simulink model "SISO_up_plant_PI_LEAD_2019a"  (R2023b)
settings: Solver=ode4  StartTime=0.0  StopTime=sim_time  FixedStep=STEP_SIZE  RelTol=1e-3  EnableMultiTasking=on
values from neighbouring files (symbols this model uses):
  A = [0 1 0 ... (first row only)    [LuenbergerObserver.m]    (also in SISO_up_plant_init.m = 0.01)
  a2 = 110544599.2    [params_aaa_elb.mat]
  b2 = 0.0564    [params_aaa_elb.mat]
  bias = -0.02    [SISO_up_plant_init.m]
  cm2m = 0.01    [params_aaa_elb.mat]
  f2 = -880    [params_aaa_elb.mat]
  freq = 1    [SISO_up_plant_init.m]
  g = 9.816    [params_aaa_elb.mat]
  g2 = 3.66    [params_aaa_elb.mat]
  h2 = 2e-05    [params_aaa_elb.mat]
  Kc_neg = 0.114    [params_aaa_elb.mat]
  Kc_pos = 0.145    [params_aaa_elb.mat]
  Kp = 6.4782e+05    (= 647820)    [SISO_up_plant_init.m]
  Kv = 5.8    [params_aaa_elb.mat]
  m = 0.1203    [params_aaa_elb.mat]
  N = 4    [params_aaa_elb.mat]
  ref = -0.02    [SISO_up_plant_init.m]
  SatLimLower = -14000    [params_aaa_elb.mat]
  SatLimUpper = 14000    [params_aaa_elb.mat]
  yc = 0.129    [params_aaa_elb.mat]
undefined symbols (not defined in the file or in its folder): den_CD, den_CPI, num_CD, num_CPI
settings Model: SimulationMode=external  Creator=s214680  LastModifiedBy=amaln
settings SolverCC: AlgebraicLoopSolver=TrustRegion
settings HardwareCC: ProdBitPerLong=64  ProdHWDeviceType=Intel->x86-64 (Linux 64)
settings SFSimCC: CustomCodeUndefinedFunction=UseInterfaceOnly
settings RTWCC: Description=Simulink Desktop Real-Time  SystemTargetFile=sldrt.tlc  TemplateMakefile=sldrt.tmf  RTWCompilerOptimization=on
settings CodeAppCC: MaxIdLength=95
settings SimulinkDesktopRealTimeCC: TargetLibSuffix=_sldrt.a  TargetPreCompLibLocation=C:\Program Files\MATLAB\R2023b\toolbox\sldrt\lib\win64  TargetLangStandard=C89/C90 (ANSI)

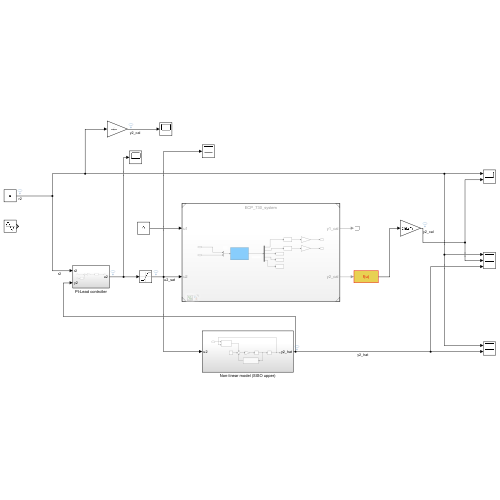
[thumbnail: Simulink's stored preview of the top-level diagram]
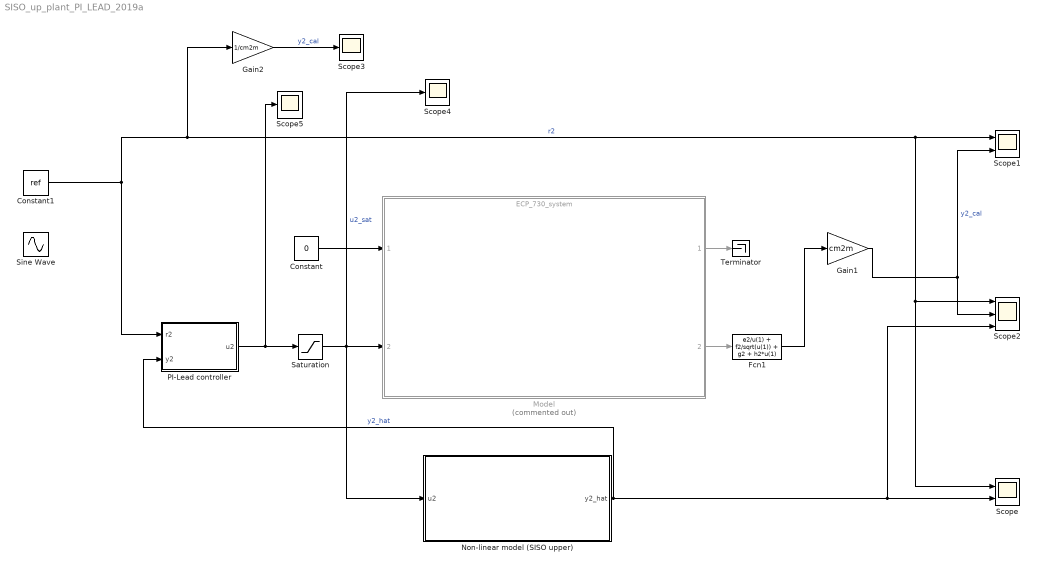
== system SISO_up_plant_PI_LEAD_2019a ==
  Constant : Constant  Value=0
  Constant1 : Constant  Value=ref  SampleTime=Inf
  Fcn1 : Fcn  Expr=e2/u(1) + f2/sqrt(u(1)) + g2 + h2*u(1)
  Gain1 : Gain  Gain=cm2m
  Gain2 : Gain  Gain=1/cm2m
  Model : ModelReference  Commented=on  ModelNameDialog=ECP_730_system  SimulationMode=Normal  ModelReferenceVersion=1.239
  Non-linear model (SISO upper) : Subsystem
  PI-Lead controller : Subsystem
  Saturation : Saturate  UpperLimit=SatLimUpper  LowerLimit=SatLimLower
  Scope : Scope  NumInputPorts=2
  Scope1 : Scope  NumInputPorts=2
  Scope2 : Scope  NumInputPorts=3
  Scope3 : Scope
  Scope4 : Scope
  Scope5 : Scope
  Sine Wave : Sin  Amplitude=A  Bias=bias  Frequency=freq  SampleTime=0
  Terminator : Terminator
  wires:
  Saturation/1 -> Non-linear model (SISO upper)/1(u2), Scope4/1, Model/2  "u2_sat"
  Non-linear model (SISO upper)/1(y2_hat) -> PI-Lead controller/2(y2), Scope/2, Scope2/3  "y2_hat"
  Fcn1/1 -> Gain1/1
  Gain1/1 -> Scope1/2, Scope2/2  "y2_cal"
  Constant/1 -> Model/1
  Model/1 -> Terminator/1
  Model/2 -> Fcn1/1
  Constant1/1 -> PI-Lead controller/1(r2), Gain2/1, Scope2/1, Scope/1, Scope1/1  "r2"
  Gain2/1 -> Scope3/1  "y2_cal"
  PI-Lead controller/1(u2) -> Scope5/1, Saturation/1

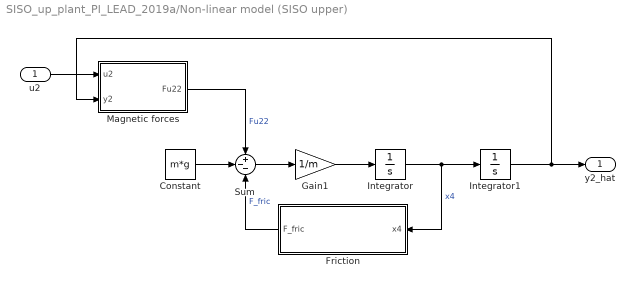
== system SISO_up_plant_PI_LEAD_2019a/Non-linear model (SISO upper) ==
  u2 : Inport
  Constant : Constant  Value=m*g
  Friction : Subsystem
  Gain1 : Gain  Gain=1/m
  Integrator : Integrator
  Integrator1 : Integrator  InitialCondition=-.03  LimitOutput=on  UpperSaturationLimit=0  LowerSaturationLimit=-yc
  Magnetic forces : Subsystem
  Sum : Sum  Inputs=+--
  y2_hat : Outport
  wires:
  Friction/1(F_fric) -> Sum/3  "F_fric"
  Constant/1 -> Sum/2
  Integrator/1 -> Integrator1/1, Friction/1(x4)  "x4"
  Gain1/1 -> Integrator/1
  Sum/1 -> Gain1/1
  Integrator1/1 -> y2_hat/1, Magnetic forces/2(y2)
  Magnetic forces/1(Fu22) -> Sum/1  "Fu22"
  u2/1 -> Magnetic forces/1(u2)

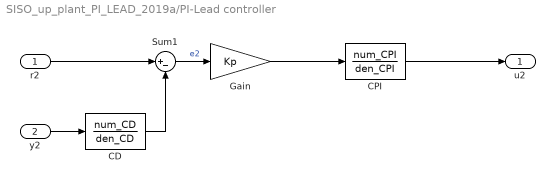
== system SISO_up_plant_PI_LEAD_2019a/PI-Lead controller ==
  r2 : Inport
  y2 : Inport  Port=2
  CD : TransferFcn  Numerator=num_CD  Denominator=den_CD
  CPI : TransferFcn  Numerator=num_CPI  Denominator=den_CPI
  Gain : Gain  Gain=Kp
  Sum1 : Sum  Inputs=|+-
  u2 : Outport
  wires:
  Sum1/1 -> Gain/1  "e2"
  r2/1 -> Sum1/1
  CPI/1 -> u2/1
  y2/1 -> CD/1
  CD/1 -> Sum1/2
  Gain/1 -> CPI/1

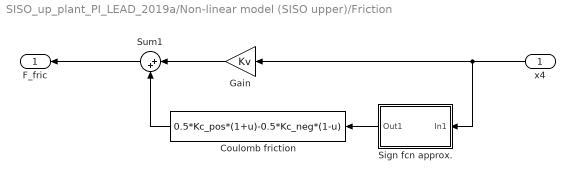
== system SISO_up_plant_PI_LEAD_2019a/Non-linear model (SISO upper)/Friction ==
  x4 : Inport
  Coulomb friction : Fcn  Expr=0.5*Kc_pos*(1+u)-0.5*Kc_neg*(1-u)
  Gain : Gain  Gain=Kv
  Sign fcn approx. : Subsystem
  Sum1 : Sum  Inputs=|++
  F_fric : Outport
  wires:
  x4/1 -> Gain/1, Sign fcn approx./1(In1)
  Sign fcn approx./1(Out1) -> Coulomb friction/1
  Gain/1 -> Sum1/1
  Coulomb friction/1 -> Sum1/2
  Sum1/1 -> F_fric/1

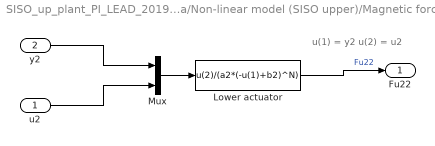
== system SISO_up_plant_PI_LEAD_2019a/Non-linear model (SISO upper)/Magnetic forces ==
  note: u(1) = y2
      | u(2) = u2
  u2 : Inport
  y2 : Inport  Port=2
  Lower actuator : Fcn  Expr=u(2)/(a2*(-u(1)+b2)^N)
  Mux : Mux  Inputs=2
  Fu22 : Outport
  wires:
  Mux/1 -> Lower actuator/1
  y2/1 -> Mux/1
  u2/1 -> Mux/2
  Lower actuator/1 -> Fu22/1  "Fu22"

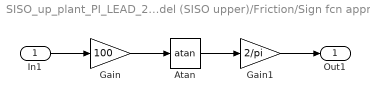
== system SISO_up_plant_PI_LEAD_2019a/Non-linear model (SISO upper)/Friction/Sign fcn approx. ==
  In1 : Inport
  Atan : Trigonometry  Operator=atan
  Gain : Gain  Gain=100
  Gain1 : Gain  Gain=2/pi
  Out1 : Outport
  wires:
  In1/1 -> Gain/1
  Gain/1 -> Atan/1
  Atan/1 -> Gain1/1
  Gain1/1 -> Out1/1
